simulink model "VCU_SW_2020"  (R2020b)
settings: Solver=FixedStepDiscrete  StartTime=0.0  StopTime=inf  FixedStep=1e-2  RelTol=1e-3
PreLoadFcn:
  | RTWConfigurationCB('preloadfcn', bdroot);
InitFcn:
  | loadvar_ttc500
undefined symbols (not defined in the file): BrkPedalTypes, CabMovModeTypes, cFuseTempSensAcc_X, cFuseTempSensAcc_Y, cFuseTempSensVal_X, cFuseTempSensVal_Y, cTMSTempSensVal_X, cTMSTempSensVal_Y, cTransferCaseSpeedRatio, diag_state, DoorsPositionTypes, dP_filter_Y, DriverOccClassSystemTypes, ErrorValueTypes, fatal_error_callback, IO_ADC_NO_RANGE, LadderStatusTypes, pAnalogCabRotSensAcc, pAnalogCabRotSensMaxVolt, pAnalogCabRotSensMinVolt, pAnalogCabRotSensRange, pAnalogCabRotSensZeroVolt, pBrkActivePress, pCabTiltSensAcc, pCabTiltSensMaxCur, pCabTiltSensMinCur, pDistanceCorrection, pECANManual_BPNEnable, pECANManual_BPNEnabler_Flag, pFilterSensAccRes, pHDirMaxDiffFrq, pHDirSensHighLvl, pHDirSensLowLvl, pMainGearRatio, pMaxFilterSensRes, pMaxFirstPedalSensValue, pMaxFuseTempSensRes, pMaxPressLoss, pMaxPressSensCurrent, pMaxPressValue, pMaxPressValueHydMotAndPump, pMaxPressValueParkDrain, pMaxSecondPedalSensValue, pMaxTempSensVoltage, pMaxTempValue, pMaxTMSTempSensRes, pMinFilterSensRes, pMinFirstPedalSensValue, pMinFuseTempSensRes, pMinPressLoss, pMinPressSensCurrent, pMinPressValue, pMinSecondPedalSensValue, pMinTempSensVoltage, pMinTempValue, pMinTMSTempSensRes, pMotorRingTeethNum, pPedalSensAccuracyPct, pPedalSensAccuracyVolt, pPressLossTreshhold ... (+20)
libraries: TTlibrary x270, canmsglib x127, simulink x88
(part 17 of 17)

== matlab function VCU_SW_2020/logSignal/getListData/listData_mf ==
  data: page input; data output; list input; len output
function [data,len] = getListDataFcn(page, list)

    data = uint8(zeros(1,7));
    len = uint8(0);

    if page == uint8(1)
        [data,len] = pageRawInput(list);
    elseif page == uint8(2)
        %data = pageInputFcns(list);
    elseif page == uint8(3)
        [data,len] = pageHighvoltageAppData(list);
    elseif page == uint8(4)
        data = pageOutputRawData(list);
    end

end

== matlab function VCU_SW_2020/logSignal/getListData/pageOutputRawData/MATLAB Function ==
  data: list input; data output
function data = fcn(list)

    data = uint8(zeros(1,7));
    if list == uint8(1)
        data = getListDataOI1();
    elseif list == uint8(2)
        data = getListDataOI2();
    elseif list == uint8(3)
        data = getListDataOI3();    
    end
end

== matlab function VCU_SW_2020/logSignal/getListData/pageRawInput/MATLAB Function ==
  data: list input; data output; len output
function [data,len] = fcn(list)
    len = uint8(0);
    data = uint8(zeros(1,7));
    if list == uint8(1)
        [data,len] = getListDataII1();
    elseif list == uint8(2)
        [data,len] = getListDataII2();
    elseif list == uint8(3)
        [data,len] = getListDataII3();    
    elseif list == uint8(4)
        [data,len] = getListDataII4();        
    elseif list == uint8(5)
        [data,len] = getListDataII5();            
    elseif list == uint8(6)
        [data,len] = getListDataII6();
    elseif list == uint8(7)
        [data,len] = getListDataII7();
    elseif list == uint8(8)
        [data,len] = getListDataII8();
    end
end

== matlab function VCU_SW_2020/logSignal/getListNum/MATLAB Function ==
  data: pageNum input; numList output
function numList = fcn(pageNum)
    numList = uint8(0);
    if pageNum == uint8(1)
        numList = uint8(8);
    elseif pageNum == uint8(2)
        numList = uint8(0);
    elseif pageNum == uint8(3)
        numList = uint8(12);
    elseif pageNum == uint8(4)
        numList = uint8(0);
    elseif pageNum == uint8(5)
        numList = uint8(3);
    end
end

== matlab function VCU_SW_2020/logSignal/getListData/pageHighvoltageAppData/MATLAB Function ==
  data: list input; data output; len output
function [data,len] = fcn(list)
len = uint8(0);
data = uint8(zeros(1,7));
if list == uint8(1)
    [data,len] = getListDataII1();
elseif list == uint8(2)
    [data,len] = getListDataII2();
elseif list == uint8(3)
    [data,len] = getListDataII3();
elseif list == uint8(4)
    [data,len] = getListDataII4();
elseif list == uint8(5)
    [data,len] = getListDataII5();
elseif list == uint8(6)
    [data,len] = getListDataII6();
elseif list == uint8(7)
    [data,len] = getListDataII7();
elseif list == uint8(8)
    [data,len] = getListDataII8();
elseif list == uint8(9)
    [data,len] = getListDataII9();
elseif list == uint8(10)
    [data,len] = getListDataII10();
elseif list == uint8(11)
    [data,len] = getListDataII11();
elseif list == uint8(12)
    [data,len] = getListDataII12();
end
end

== matlab function VCU_SW_2020/ServerFcn/convINint16/MATLAB Function2 ==
  data: x input; y output
function y = fcn(x)

y = int16(x);

end

== matlab function VCU_SW_2020/ServerFcn/convINuint16/MATLAB Function2 ==
  data: x input; y output
function y = fcn(x)

y = uint16(x);

end

== matlab function VCU_SW_2020/EEPROM Layer/calculate trip distance/calcTripDist ==
  data: vehSpd input; distance output; correction input; a output
function [distance, a] = calcDist(vehSpd, correction)

vehSpdInMS = single(vehSpd) * single(0.28);
persistent exSpd cnt exDist exDistSum
if isempty(exSpd)
    exSpd = vehSpdInMS;
    cnt = uint8(0);
    exDist = single(0);
    exDistSum = single(0);
end


if cnt < uint8(10)
    cnt = cnt + uint8(1);
    distance = uint32(0);
else
    cnt = uint8(0);
    exDist = (single((vehSpdInMS + exSpd)) * single(0.5) * single(0.1)) * correction;
    exSpd = vehSpdInMS;
    if exDist >= single(1)
        distance = uint32(exDist);
        exDistSum = single(0);
    else
        if exDistSum >= single(1)
            distance = uint32(exDistSum);
            exDistSum = single(0);
        else
            exDistSum = exDistSum + exDist;
            distance = uint32(0);
        end
    end
end

a = (single((vehSpdInMS + exSpd)) * single(0.5) * single(0.1));

end

== matlab function VCU_SW_2020/EEPROM Layer/calculate trip distance/EEPROM read/calcTotalDist ==
  data: tripDist input; updDistM output; savedDistM input; savedDistKM input; savedDistKKM input; updDistKM output; updDistKKM output; updDistTotal output
function [updDistM, updDistKM, updDistKKM, updDistTotal] = calcTotalDist(tripDist, ...
    savedDistM, savedDistKM, savedDistKKM)

updDistTotal = tripDist ...
    + uint32(savedDistKKM) * uint32(1000000) ...
    + uint32(savedDistKM) * uint32(1000) ...
    + uint32(savedDistM);

if uint16((updDistTotal - uint32(500000)) / uint32(1000000)) < uint16(1000)
    updDistKKM = uint16((updDistTotal - uint32(500000)) / uint32(1000000));
else
   updDistKKM = uint16(0);
end

updDistKM = uint16((uint32(updDistTotal - uint32(updDistKKM) ...
    * uint32(1000000)) - uint32(500)) / uint32(1000));

updDistM = uint16(updDistTotal - uint32(updDistKKM) * ...
    uint32(1000000) - uint32(updDistKM) * uint32(1000));

end

== matlab function VCU_SW_2020/InputLayer/InputNetwork/InputCCAN/CCAN100msecProc1/JoystickRot/MATLAB Function ==
  data: neutralPos input; fwdPos input; bckwsPos input; absPos input; pos output; dir output
function [pos, dir] = fcn(neutralPos, fwdPos, bckwsPos, absPos)

    if absPos > single(100)
        pos = uint8(100);
    else
        pos = uint8(absPos);
    end

    if fwdPos == 1 &&...
       bckwsPos == 0
        dir = CabRotDirTypes.ROT_RIGHT;
    elseif fwdPos == 0 &&...
           bckwsPos == 1
        dir = CabRotDirTypes.ROT_LEFT;
    elseif neutralPos == 1
        dir = CabRotDirTypes.ROT_STANDBY;
    else
        dir = CabRotDirTypes.ROT_NOT_DEFINED;
        pos = uint8(0);
    end

end

== matlab function VCU_SW_2020/EEPROM Layer/Simulink Function1/eeprom_write_processing_kora ==
  data: UDSStruct data_store_memory; flag output; write_sts output
function [flag, write_sts] = writeProcessing()

    global UDSStruct
    
    %флаг вызова фунцкии записи
    flag = false;
    
    eeprom_write_sts = uint16(15);

    if (coder.target('MATLAB')) || (coder.target('Sfun'))

    else
        
        data = zeros(9, 1, 'uint32');
        data(1) = uint32(UDSStruct.DistanceM);
        data(2) = uint32(UDSStruct.DistanceKM);
        data(3) = uint32(UDSStruct.DistanceKKM);
        data(4) = uint32(UDSStruct.EngineHours);
        data(5) = uint32(UDSStruct.TransPumpVolumeMax);
        data(6) = uint32(UDSStruct.TransMotorVolumeMin);
        data(7) = uint32(UDSStruct.AccelerationPedalMaxEngSpd);
        data(8) = uint32(UDSStruct.AccelerationPedalMinEngSpd);
        data(9) = uint32(UDSStruct.EngineSpeedMax);
        data(10) = uint32(UDSStruct.EngineSpeedMin);
        
        %Вызов функции перекладывания данных в буфер EEPROM
        coder.ceval('put_EEPROM_data', data);
        eeprom_write_sts = coder.ceval('get_writeSts');
        %Выставление флага записи в буфер
        coder.ceval('set_write_flag', uint8(1));
                
        flag = true;
        
    end
    
    write_sts = eeprom_write_sts;
    
end
